simulink model "CryoDetMultiChan_CMB"  (R2016b)
settings: Solver=ode45  StartTime=0.0  StopTime=400e-6  MaxStep=Tclk/4  RelTol=1e-3
values from neighbouring files (symbols this model uses):
  ds_axi = 16    [setupCryoFPGA_CMB.m]
  Fclk = Fadc    (= 307200000)    [setupCryoFPGA_CMB.m]
  lpf = tf(num,den)    [setupCryoFPGA_CMB.m]
  Tclk = 1/Fclk    (= 3.25520833333e-09)    [setupCryoFPGA_CMB.m]
  Ts = 1/Fs    (= 3.25520833333e-09)    [setupADCtoDACloopback.m]    (also in setupCryoFPGA_CMB.m)
undefined symbols (not defined in the file or in its folder): AXI4, i, Lite, xlipgetpartsetting
libraries: xbsIndex_r4 x2215, hdlsllib x6, simulink x3, CryoDetLib x2
(part 16 of 16)

== system CryoDetMultiChan_CMB/DspCore/FTA_Ch0/loopFilter/initial Frequencies ==
  note: Channel 15 used for none of above
  note: initial Frequencies
  note: select initial frequency
      | for now just mux from input registers
      | eventually configure RAM and loading protocol
  channel : Inport
  BitBasher : xbsIndex_r4/BitBasher  bitexpr=a={b[3:0]}  display_expr=off  sr_1=a  arith_type1=Unsigned  bin_pt1=0  sr_2=2  arith_type2=Unsigned  bin_pt2=0  sr_3=3  arith_type3=Unsigned  bin_pt3=0  sr_4=4  arith_type4=Unsigned  bin_pt4=0  dbl_ovrd=off  block_type=bitbasher
  Gateway Out12 : xbsIndex_r4/Gateway Out  inherit_from_input=off  hdl_port=off  rows=1  columns=1  UseAsDAC=off  DACChannel='1'  interface=None  automatic_assignment=on  address_offset=hex2dec('00')  intf_name=''  intf_description=''  timing_constraint=None  locs_specified=off  LOCs={}  io_standard={}  block_type=gatewayout
  Gateway Out13 : xbsIndex_r4/Gateway Out  inherit_from_input=off  hdl_port=off  rows=1  columns=1  UseAsDAC=off  DACChannel='1'  interface=None  automatic_assignment=on  address_offset=hex2dec('00')  intf_name=''  intf_description=''  timing_constraint=None  locs_specified=off  LOCs={}  io_standard={}  block_type=gatewayout
  Mux : xbsIndex_r4/Mux  inputs=16  en=off  latency=0  precision=Full  arith_type=Unsigned  n_bits=24  bin_pt=24  quantization=Truncate  overflow=Wrap  dbl_ovrd=off  block_type=mux
  initial Freqs : Scope  NumInputPorts=2
  Fi : Outport
  wires:
  BitBasher/1 -> Mux/1, Gateway Out12/1
  [F0] -> Mux/2
  [F1] -> Mux/3
  [F2] -> Mux/4
  [F3] -> Mux/5
  [F4] -> Mux/6
  [F5] -> Mux/7
  [F6] -> Mux/8
  [F7] -> Mux/9
  [F8] -> Mux/10
  [F9] -> Mux/11
  [F10] -> Mux/12
  [F11] -> Mux/13
  Mux/1 -> Gateway Out13/1, Fi/1
  Gateway Out13/1 -> initial Freqs/2
  Gateway Out12/1 -> initial Freqs/1
  [F12] -> Mux/14
  [F13] -> Mux/15
  [F14] -> Mux/16
  [F15] -> Mux/17
  channel/1 -> BitBasher/1

== system CryoDetMultiChan_CMB/DspCore/FTA_Ch0/SixteenLineUDC 0/DAC Sum1/DAC UC I sum ==
  note: Changed from 12 channel to 16 channels 8Sept2017
  note: Final adder stages
      | divide by 8
      | and reduce to 16 bits
  In1 : Inport
  AddSub{,2,4,6,8,10,12..15,24..27} (14 alike) : xbsIndex_r4/AddSub  mode=Addition  use_carryin=off  use_carryout=off  en=off  latency=3  precision=User Defined  arith_type="Signed  (2's comp)"  n_bits=20  bin_pt=15  quantization=Truncate  overflow=Wrap  use_behavioral_HDL=off  hw_selection=Fabric  pipelined=off  dbl_ovrd=off  block_type=addsub
  AddSub20 : xbsIndex_r4/AddSub  mode=Addition  use_carryin=off  use_carryout=off  en=off  latency=3  precision=User Defined  arith_type="Signed  (2's comp)"  n_bits=16  bin_pt=15  quantization="Round  (unbiased: +/- Inf)"  overflow=Saturate  use_behavioral_HDL=off  hw_selection=Fabric  pipelined=off  dbl_ovrd=off  block_type=addsub
  Bus Selector1 : BusSelector  OutputSignals=UC_out_line15.UC_out_I,UC_out_line14.UC_out_I,UC_out_line13.UC_out_I,UC_out_line12.UC_out_I,UC_out_line11.UC_out_I,UC_out_line10.UC_out_I,UC_out_line9.UC_out_I,UC_out_line8.UC_out_I,UC_out_line7.UC_out_I,UC_out_line6.UC_out_I,UC_out_line5.UC_out_I,UC_out_line4.UC_out_I,UC_out_line3.UC_out_I,UC_out_line2.UC_out_I,UC_out_line1.UC_out_I,UC_out_line0.UC_out_I
  DAC subSum scope : Scope  NumInputPorts=2
  Gateway Out : xbsIndex_r4/Gateway Out  inherit_from_input=off  hdl_port=off  rows=1  columns=1  UseAsDAC=off  DACChannel='1'  interface=None  automatic_assignment=on  address_offset=hex2dec('00')  intf_name=''  intf_description=''  timing_constraint=None  locs_specified=off  LOCs={}  io_standard={}  block_type=gatewayout
  Gateway Out1 : xbsIndex_r4/Gateway Out  inherit_from_input=off  hdl_port=off  rows=1  columns=1  UseAsDAC=off  DACChannel='1'  interface=None  automatic_assignment=on  address_offset=hex2dec('00')  intf_name=''  intf_description=''  timing_constraint=None  locs_specified=off  LOCs={}  io_standard={}  block_type=gatewayout
  Scale : xbsIndex_r4/Scale  scale_factor=-3  dbl_ovrd=off  block_type=scale
  Scale1 : xbsIndex_r4/Scale  scale_factor=-3  dbl_ovrd=off  block_type=scale
  Out1 : Outport
  wires:
  In1/1 -> Bus Selector1/1
  AddSub20/1 -> Out1/1
  AddSub/1 -> AddSub12/1
  AddSub2/1 -> AddSub12/2
  AddSub4/1 -> AddSub13/1
  AddSub6/1 -> AddSub13/2
  AddSub8/1 -> AddSub14/1
  AddSub10/1 -> AddSub14/2
  AddSub12/1 -> AddSub15/1
  AddSub13/1 -> AddSub15/2
  AddSub15/1 -> Scale/1
  Bus Selector1/1 -> AddSub/1  "<UC_out_I>"
  Scale/1 -> Gateway Out/1, AddSub20/1
  Scale1/1 -> Gateway Out1/1, AddSub20/2
  AddSub25/1 -> AddSub26/1
  AddSub24/1 -> AddSub26/2
  AddSub14/1 -> AddSub27/1
  AddSub27/1 -> Scale1/1
  AddSub26/1 -> AddSub27/2
  Bus Selector1/16 -> AddSub24/2  "<UC_out_I>"
  Bus Selector1/15 -> AddSub24/1  "<UC_out_I>"
  Bus Selector1/14 -> AddSub25/2  "<UC_out_I>"
  Bus Selector1/13 -> AddSub25/1  "<UC_out_I>"
  Bus Selector1/12 -> AddSub10/2  "<UC_out_I>"
  Bus Selector1/11 -> AddSub10/1  "<UC_out_I>"
  Bus Selector1/10 -> AddSub8/2  "<UC_out_I>"
  Bus Selector1/9 -> AddSub8/1  "<UC_out_I>"
  Bus Selector1/7 -> AddSub6/1  "<UC_out_I>"
  Bus Selector1/6 -> AddSub4/2  "<UC_out_I>"
  Bus Selector1/5 -> AddSub4/1  "<UC_out_I>"
  Bus Selector1/4 -> AddSub2/2  "<UC_out_I>"
  Bus Selector1/3 -> AddSub2/1  "<UC_out_I>"
  Bus Selector1/2 -> AddSub/2  "<UC_out_I>"
  Bus Selector1/8 -> AddSub6/2  "<UC_out_I>"
  Gateway Out1/1 -> DAC subSum scope/2
  Gateway Out/1 -> DAC subSum scope/1

== system CryoDetMultiChan_CMB/DspCore/FTA_Ch0/SixteenLineUDC 0/DAC Sum1/DAC UC Q sum ==
  note: Changed from 12 channel to 16 channels 8Sept2017
  note: Final adder stages
      | divide by 8
      | and reduce to 16 bits
  In1 : Inport
  AddSub{,2,4,6,8,10,12..15,24..27} (14 alike) : xbsIndex_r4/AddSub  mode=Addition  use_carryin=off  use_carryout=off  en=off  latency=3  precision=User Defined  arith_type="Signed  (2's comp)"  n_bits=20  bin_pt=15  quantization=Truncate  overflow=Wrap  use_behavioral_HDL=off  hw_selection=Fabric  pipelined=off  dbl_ovrd=off  block_type=addsub
  AddSub20 : xbsIndex_r4/AddSub  mode=Addition  use_carryin=off  use_carryout=off  en=off  latency=3  precision=User Defined  arith_type="Signed  (2's comp)"  n_bits=16  bin_pt=15  quantization="Round  (unbiased: +/- Inf)"  overflow=Saturate  use_behavioral_HDL=off  hw_selection=Fabric  pipelined=off  dbl_ovrd=off  block_type=addsub
  Bus Selector1 : BusSelector  OutputSignals=UC_out_line15.UC_out_Q,UC_out_line14.UC_out_Q,UC_out_line13.UC_out_Q,UC_out_line12.UC_out_Q,UC_out_line11.UC_out_Q,UC_out_line10.UC_out_Q,UC_out_line9.UC_out_Q,UC_out_line8.UC_out_Q,UC_out_line7.UC_out_Q,UC_out_line6.UC_out_Q,UC_out_line5.UC_out_Q,UC_out_line4.UC_out_Q,UC_out_line3.UC_out_Q,UC_out_line2.UC_out_Q,UC_out_line1.UC_out_Q,UC_out_line0.UC_out_Q
  DAC subSum scope : Scope  NumInputPorts=2
  Gateway Out : xbsIndex_r4/Gateway Out  inherit_from_input=off  hdl_port=off  rows=1  columns=1  UseAsDAC=off  DACChannel='1'  interface=None  automatic_assignment=on  address_offset=hex2dec('00')  intf_name=''  intf_description=''  timing_constraint=None  locs_specified=off  LOCs={}  io_standard={}  block_type=gatewayout
  Gateway Out1 : xbsIndex_r4/Gateway Out  inherit_from_input=off  hdl_port=off  rows=1  columns=1  UseAsDAC=off  DACChannel='1'  interface=None  automatic_assignment=on  address_offset=hex2dec('00')  intf_name=''  intf_description=''  timing_constraint=None  locs_specified=off  LOCs={}  io_standard={}  block_type=gatewayout
  Scale : xbsIndex_r4/Scale  scale_factor=-3  dbl_ovrd=off  block_type=scale
  Scale1 : xbsIndex_r4/Scale  scale_factor=-3  dbl_ovrd=off  block_type=scale
  Out1 : Outport
  wires:
  In1/1 -> Bus Selector1/1
  AddSub20/1 -> Out1/1
  AddSub/1 -> AddSub12/1
  AddSub2/1 -> AddSub12/2
  AddSub4/1 -> AddSub13/1
  AddSub6/1 -> AddSub13/2
  AddSub8/1 -> AddSub14/1
  AddSub10/1 -> AddSub14/2
  AddSub12/1 -> AddSub15/1
  AddSub13/1 -> AddSub15/2
  AddSub15/1 -> Scale/1
  Bus Selector1/1 -> AddSub/1  "<UC_out_Q>"
  Scale/1 -> Gateway Out/1, AddSub20/1
  Scale1/1 -> Gateway Out1/1, AddSub20/2
  AddSub25/1 -> AddSub26/1
  AddSub24/1 -> AddSub26/2
  AddSub14/1 -> AddSub27/1
  AddSub27/1 -> Scale1/1
  AddSub26/1 -> AddSub27/2
  Bus Selector1/16 -> AddSub24/2  "<UC_out_Q>"
  Bus Selector1/15 -> AddSub24/1  "<UC_out_Q>"
  Bus Selector1/14 -> AddSub25/2  "<UC_out_Q>"
  Bus Selector1/13 -> AddSub25/1  "<UC_out_Q>"
  Bus Selector1/12 -> AddSub10/2  "<UC_out_Q>"
  Bus Selector1/11 -> AddSub10/1  "<UC_out_Q>"
  Bus Selector1/10 -> AddSub8/2  "<UC_out_Q>"
  Bus Selector1/9 -> AddSub8/1  "<UC_out_Q>"
  Bus Selector1/7 -> AddSub6/1  "<UC_out_Q>"
  Bus Selector1/6 -> AddSub4/2  "<UC_out_Q>"
  Bus Selector1/5 -> AddSub4/1  "<UC_out_Q>"
  Bus Selector1/4 -> AddSub2/2  "<UC_out_Q>"
  Bus Selector1/3 -> AddSub2/1  "<UC_out_Q>"
  Bus Selector1/2 -> AddSub/2  "<UC_out_Q>"
  Bus Selector1/8 -> AddSub6/2  "<UC_out_Q>"
  Gateway Out1/1 -> DAC subSum scope/2
  Gateway Out/1 -> DAC subSum scope/1

== system CryoDetMultiChan_CMB/DspCore/FTA_Ch0/SixteenLineUDC 0/DAC Sum1/DAC UC Qi sum ==
  note: Changed from 12 channel to 16 channels 8Sept2017
  note: Final adder stages
      | divide by 8
      | and reduce to 16 bits
  In1 : Inport
  AddSub{,2,4,6,8,10,12..15,24..27} (14 alike) : xbsIndex_r4/AddSub  mode=Addition  use_carryin=off  use_carryout=off  en=off  latency=3  precision=User Defined  arith_type="Signed  (2's comp)"  n_bits=20  bin_pt=15  quantization=Truncate  overflow=Wrap  use_behavioral_HDL=off  hw_selection=Fabric  pipelined=off  dbl_ovrd=off  block_type=addsub
  AddSub20 : xbsIndex_r4/AddSub  mode=Addition  use_carryin=off  use_carryout=off  en=off  latency=3  precision=User Defined  arith_type="Signed  (2's comp)"  n_bits=16  bin_pt=15  quantization="Round  (unbiased: +/- Inf)"  overflow=Saturate  use_behavioral_HDL=off  hw_selection=Fabric  pipelined=off  dbl_ovrd=off  block_type=addsub
  Bus Selector1 : BusSelector  OutputSignals=UC_out_line15.UC_out_Ip,UC_out_line14.UC_out_Ip,UC_out_line13.UC_out_Ip,UC_out_line12.UC_out_Ip,UC_out_line11.UC_out_Ip,UC_out_line10.UC_out_Ip,UC_out_line9.UC_out_Ip,UC_out_line8.UC_out_Ip,UC_out_line7.UC_out_Ip,UC_out_line6.UC_out_Ip,UC_out_line5.UC_out_Ip,UC_out_line4.UC_out_Ip,UC_out_line3.UC_out_Ip,UC_out_line2.UC_out_Ip,UC_out_line1.UC_out_Ip,UC_out_line0.UC_out_Ip
  DAC subSum scope : Scope  NumInputPorts=2
  Gateway Out : xbsIndex_r4/Gateway Out  inherit_from_input=off  hdl_port=off  rows=1  columns=1  UseAsDAC=off  DACChannel='1'  interface=None  automatic_assignment=on  address_offset=hex2dec('00')  intf_name=''  intf_description=''  timing_constraint=None  locs_specified=off  LOCs={}  io_standard={}  block_type=gatewayout
  Gateway Out1 : xbsIndex_r4/Gateway Out  inherit_from_input=off  hdl_port=off  rows=1  columns=1  UseAsDAC=off  DACChannel='1'  interface=None  automatic_assignment=on  address_offset=hex2dec('00')  intf_name=''  intf_description=''  timing_constraint=None  locs_specified=off  LOCs={}  io_standard={}  block_type=gatewayout
  Scale : xbsIndex_r4/Scale  scale_factor=-3  dbl_ovrd=off  block_type=scale
  Scale1 : xbsIndex_r4/Scale  scale_factor=-3  dbl_ovrd=off  block_type=scale
  Out1 : Outport
  wires:
  In1/1 -> Bus Selector1/1
  AddSub20/1 -> Out1/1
  AddSub/1 -> AddSub12/1
  AddSub2/1 -> AddSub12/2
  AddSub4/1 -> AddSub13/1
  AddSub6/1 -> AddSub13/2
  AddSub8/1 -> AddSub14/1
  AddSub10/1 -> AddSub14/2
  AddSub12/1 -> AddSub15/1
  AddSub13/1 -> AddSub15/2
  AddSub15/1 -> Scale/1
  Bus Selector1/1 -> AddSub/1  "<UC_out_Ip>"
  Scale/1 -> Gateway Out/1, AddSub20/1
  Scale1/1 -> Gateway Out1/1, AddSub20/2
  AddSub25/1 -> AddSub26/1
  AddSub24/1 -> AddSub26/2
  AddSub14/1 -> AddSub27/1
  AddSub27/1 -> Scale1/1
  AddSub26/1 -> AddSub27/2
  Bus Selector1/16 -> AddSub24/2  "<UC_out_Ip>"
  Bus Selector1/15 -> AddSub24/1  "<UC_out_Ip>"
  Bus Selector1/14 -> AddSub25/2  "<UC_out_Ip>"
  Bus Selector1/13 -> AddSub25/1  "<UC_out_Ip>"
  Bus Selector1/12 -> AddSub10/2  "<UC_out_Ip>"
  Bus Selector1/11 -> AddSub10/1  "<UC_out_Ip>"
  Bus Selector1/10 -> AddSub8/2  "<UC_out_Ip>"
  Bus Selector1/9 -> AddSub8/1  "<UC_out_Ip>"
  Bus Selector1/7 -> AddSub6/1  "<UC_out_Ip>"
  Bus Selector1/6 -> AddSub4/2  "<UC_out_Ip>"
  Bus Selector1/5 -> AddSub4/1  "<UC_out_Ip>"
  Bus Selector1/4 -> AddSub2/2  "<UC_out_Ip>"
  Bus Selector1/3 -> AddSub2/1  "<UC_out_Ip>"
  Bus Selector1/2 -> AddSub/2  "<UC_out_Ip>"
  Bus Selector1/8 -> AddSub6/2  "<UC_out_Ip>"
  Gateway Out1/1 -> DAC subSum scope/2
  Gateway Out/1 -> DAC subSum scope/1

== system CryoDetMultiChan_CMB/DspCore/FTA_Ch0/SixteenLineUDC 0/DAC Sum1/DAC UC Qp sum ==
  note: Changed from 12 channel to 16 channels 8Sept2017
  note: Final adder stages
      | divide by 8
      | and reduce to 16 bits
  In1 : Inport
  AddSub{,2,4,6,8,10,12..15,24..27} (14 alike) : xbsIndex_r4/AddSub  mode=Addition  use_carryin=off  use_carryout=off  en=off  latency=3  precision=User Defined  arith_type="Signed  (2's comp)"  n_bits=20  bin_pt=15  quantization=Truncate  overflow=Wrap  use_behavioral_HDL=off  hw_selection=Fabric  pipelined=off  dbl_ovrd=off  block_type=addsub
  AddSub20 : xbsIndex_r4/AddSub  mode=Addition  use_carryin=off  use_carryout=off  en=off  latency=3  precision=User Defined  arith_type="Signed  (2's comp)"  n_bits=16  bin_pt=15  quantization="Round  (unbiased: +/- Inf)"  overflow=Saturate  use_behavioral_HDL=off  hw_selection=Fabric  pipelined=off  dbl_ovrd=off  block_type=addsub
  Bus Selector1 : BusSelector  OutputSignals=UC_out_line15.UC_out_Qp,UC_out_line14.UC_out_Qp,UC_out_line13.UC_out_Qp,UC_out_line12.UC_out_Qp,UC_out_line11.UC_out_Qp,UC_out_line10.UC_out_Qp,UC_out_line9.UC_out_Qp,UC_out_line8.UC_out_Qp,UC_out_line7.UC_out_Qp,UC_out_line6.UC_out_Qp,UC_out_line5.UC_out_Qp,UC_out_line4.UC_out_Qp,UC_out_line3.UC_out_Qp,UC_out_line2.UC_out_Qp,UC_out_line1.UC_out_Qp,UC_out_line0.UC_out_Qp
  DAC subSum scope : Scope  NumInputPorts=2
  Gateway Out : xbsIndex_r4/Gateway Out  inherit_from_input=off  hdl_port=off  rows=1  columns=1  UseAsDAC=off  DACChannel='1'  interface=None  automatic_assignment=on  address_offset=hex2dec('00')  intf_name=''  intf_description=''  timing_constraint=None  locs_specified=off  LOCs={}  io_standard={}  block_type=gatewayout
  Gateway Out1 : xbsIndex_r4/Gateway Out  inherit_from_input=off  hdl_port=off  rows=1  columns=1  UseAsDAC=off  DACChannel='1'  interface=None  automatic_assignment=on  address_offset=hex2dec('00')  intf_name=''  intf_description=''  timing_constraint=None  locs_specified=off  LOCs={}  io_standard={}  block_type=gatewayout
  Scale : xbsIndex_r4/Scale  scale_factor=-3  dbl_ovrd=off  block_type=scale
  Scale1 : xbsIndex_r4/Scale  scale_factor=-3  dbl_ovrd=off  block_type=scale
  Out1 : Outport
  wires:
  In1/1 -> Bus Selector1/1
  AddSub20/1 -> Out1/1
  AddSub/1 -> AddSub12/1
  AddSub2/1 -> AddSub12/2
  AddSub4/1 -> AddSub13/1
  AddSub6/1 -> AddSub13/2
  AddSub8/1 -> AddSub14/1
  AddSub10/1 -> AddSub14/2
  AddSub12/1 -> AddSub15/1
  AddSub13/1 -> AddSub15/2
  AddSub15/1 -> Scale/1
  Bus Selector1/1 -> AddSub/1  "<UC_out_Qp>"
  Scale/1 -> Gateway Out/1, AddSub20/1
  Scale1/1 -> Gateway Out1/1, AddSub20/2
  AddSub25/1 -> AddSub26/1
  AddSub24/1 -> AddSub26/2
  AddSub14/1 -> AddSub27/1
  AddSub27/1 -> Scale1/1
  AddSub26/1 -> AddSub27/2
  Bus Selector1/16 -> AddSub24/2  "<UC_out_Qp>"
  Bus Selector1/15 -> AddSub24/1  "<UC_out_Qp>"
  Bus Selector1/14 -> AddSub25/2  "<UC_out_Qp>"
  Bus Selector1/13 -> AddSub25/1  "<UC_out_Qp>"
  Bus Selector1/12 -> AddSub10/2  "<UC_out_Qp>"
  Bus Selector1/11 -> AddSub10/1  "<UC_out_Qp>"
  Bus Selector1/10 -> AddSub8/2  "<UC_out_Qp>"
  Bus Selector1/9 -> AddSub8/1  "<UC_out_Qp>"
  Bus Selector1/7 -> AddSub6/1  "<UC_out_Qp>"
  Bus Selector1/6 -> AddSub4/2  "<UC_out_Qp>"
  Bus Selector1/5 -> AddSub4/1  "<UC_out_Qp>"
  Bus Selector1/4 -> AddSub2/2  "<UC_out_Qp>"
  Bus Selector1/3 -> AddSub2/1  "<UC_out_Qp>"
  Bus Selector1/2 -> AddSub/2  "<UC_out_Qp>"
  Bus Selector1/8 -> AddSub6/2  "<UC_out_Qp>"
  Gateway Out1/1 -> DAC subSum scope/2
  Gateway Out/1 -> DAC subSum scope/1

== system CryoDetMultiChan_CMB/DspCore/FTA_Ch0/SixteenLineUDC 0/DC_decimate/CIC reset ==
  note: where N is number of channels in CIC filter
  note: reset latched resetIn
  note: latch resetIn
  note: CIC reset
      |
      | Synchronizes a CIC compiler 4.0 multi-channel CIC filter
      | to input channels
      |
      | Generates:
      | 1	notResetOut to CIC aresetn
      | 2	tlast to CIC tlast input
      |
      | Inputs:
      | 1	reset in
      | 2	Channel number (0-N) which may go to sel input of mux generating the input data stream
      | 3	N-2 which tells this module how deep is the multiplexing (e.g. N-2 = 10 for a 12 channel CIC filter (sorry))
      |
      | Guarantees:
      | 1	reset out is at least 2 clocks long
      | 2	end of reset occurs 2 clocks before channel 0
      | 3	tlast comes with channel N-1
      |
      | Assumes:
      | CIC oversampling set to "Sample period" = 1
      | No "streaming interface"
  resetIn : Inport
  Channel : Inport  Port=2
  N-2 : Inport  Port=3
  Constant : xbsIndex_r4/Constant  const=0  gui_display_data_type=Boolean  arith_type=Boolean  n_bits=16  bin_pt=14  preci_type=Single  exp_width=8  frac_width=24  explicit_period=off  period=1  equ=P=C  opselect=C  inp2=PCIN>>17  opr=+  inp1=P  carry=CIN  dbl_ovrd=off  block_type=constant
  Delay1 : xbsIndex_r4/Delay  rst=off  infoeditControl=Selection of Reset will increase slice count due to use of real FFs and instead of SRLs  en=off  latency=1  reg_retiming=off  dbl_ovrd=off  block_type=delay
  Delay2 : xbsIndex_r4/Delay  rst=off  infoeditControl=Selection of Reset will increase slice count due to use of real FFs and instead of SRLs  en=off  latency=1  reg_retiming=off  dbl_ovrd=off  block_type=delay
  Delay3 : xbsIndex_r4/Delay  rst=off  infoeditControl=Selection of Reset will increase slice count due to use of real FFs and instead of SRLs  en=off  latency=1  reg_retiming=off  dbl_ovrd=off  block_type=delay
  Inverter : xbsIndex_r4/Inverter  en=off  latency=2  dbl_ovrd=off  block_type=inv
  Inverter1 : xbsIndex_r4/Inverter  en=off  latency=0  dbl_ovrd=off  block_type=inv
  Logical : xbsIndex_r4/Logical  logical_function=AND  inputs=4  en=off  latency=0  precision=User Defined  arith_type=Boolean  n_bits=1  bin_pt=0  align_bp=on  dbl_ovrd=off  block_type=logical
  Logical1 : xbsIndex_r4/Logical  logical_function=OR  inputs=2  en=off  latency=0  precision=User Defined  arith_type=Boolean  n_bits=1  bin_pt=0  align_bp=on  dbl_ovrd=off  block_type=logical
  Mux : xbsIndex_r4/Mux  inputs=2  en=off  latency=0  precision=Full  arith_type=Unsigned  n_bits=16  bin_pt=14  quantization=Truncate  overflow=Wrap  dbl_ovrd=off  block_type=mux
  Relational1 : xbsIndex_r4/Relational  mode=a=b  op_type=Bool  en=off  latency=0  dbl_ovrd=off  block_type=relational
  notResetOut : Outport
  tlast : Outport  Port=2
  wires:
  resetIn/1 -> Inverter/1, Logical1/1
  Channel/1 -> Relational1/1
  N-2/1 -> Relational1/2
  Relational1/1 -> Logical/4, Delay1/1
  Logical1/1 -> Inverter1/1, Delay2/1
  Mux/1 -> Logical1/2
  Delay2/1 -> Logical/2, Delay3/1, Mux/2
  Constant/1 -> Mux/3
  Logical/1 -> Mux/1
  Delay1/1 -> tlast/1
  Inverter/1 -> Logical/1
  Delay3/1 -> Logical/3
  Inverter1/1 -> notResetOut/1
